simulink model "Ir test"  (R2022a)
settings: Solver=ode3  StartTime=0.0  StopTime=inf  RelTol=1e-3  EnableMultiTasking=on
settings Model: ExtModeTrigDuration=25  Creator=The MathWorks, Inc.  LastModifiedBy=impre
settings SolverCC: AlgebraicLoopSolver=TrustRegion
settings DataIOCC: LimitDataPoints=on  SaveFormat=Array  ReturnWorkspaceOutputs=off
settings OptimizationCC: ExpressionDepthLimit=2147483647  LifeSpan=Inf  MaxStackSize=64
settings DebuggingCC: UnderspecifiedInitializationDetection=Classic  MergeDetectMultiDrivingBlocksExec=none  InheritedTsInSrcMsg=none  FcnCallInpInsideContextMsg=warning  UnconnectedLineMsg=warning  AllowSymbolicDim=off  StateNameClashWarn=warning  SFUnexpectedBacktrackingDiag=warning  SFNoUnconditionalDefaultTransitionDiag=warning  SFExecutionAtInitializationDiag=none  SFMachineParentedDataDiag=warning  ArithmeticOperatorsInVariantConditions=warning
settings HardwareCC: ProdBitPerPointer=32  ProdBitPerSizeT=32  ProdBitPerPtrDiffT=32  ProdLargestAtomicInteger=Long  ProdLargestAtomicFloat=Double  ProdWordSize=32  ProdHWDeviceType=ARM Compatible->ARM Cortex  UseEmbeddedCoderFeatures=off
settings ModelReferenceCC: PropagateSignalLabelsOutOfModel=off
settings SFSimCC: SimUseLocalCustomCode=off  CustomCodeUndefinedFunction=UseInterfaceOnly
settings RTWCC: SystemTargetFile=ert.tlc  HardwareBoard=ARM Cortex-based VEX Microcontroller  TLCOptions=-aInlineSetEventsForThisBaseRateFcn=TLC_FALSE -aSuppressMultiTaskScheduler=TLC_FALSE -aRateBasedStepFcn=0  TemplateMakefile=ert_default_tmf  GenerateReport=on  RTWUseLocalCustomCode=off  Toolchain=GNU Tools for VEX ARM Cortex  LaunchReport=on  DLArmComputeVersion=19.05
settings CodeAppCC: StateflowObjectComments=on
settings ERTTargetCC: CodeReplacementLibrary=GCC ARM Cortex-M3  MultiwordLength=2048  ERTCustomFileBanners=off  SupportContinuousTime=on  SupportNonInlinedSFcns=on  RemoveResetFunc=off  ModelStepFunctionPrototypeControlCompliant=off  ConvertIfToSwitch=off  SuppressUnreachableDefaultCases=off
settings ConfigComp: CovMetricSettings=dw  CovSaveCumulativeToWorkspaceVar=on  CovSaveSingleToWorkspaceVar=on  CovExternalEMLEnable=off  CovSFcnEnable=off

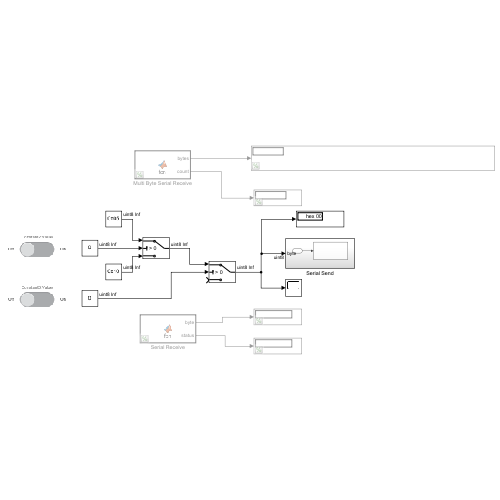
[thumbnail: Simulink's stored preview of the top-level diagram]
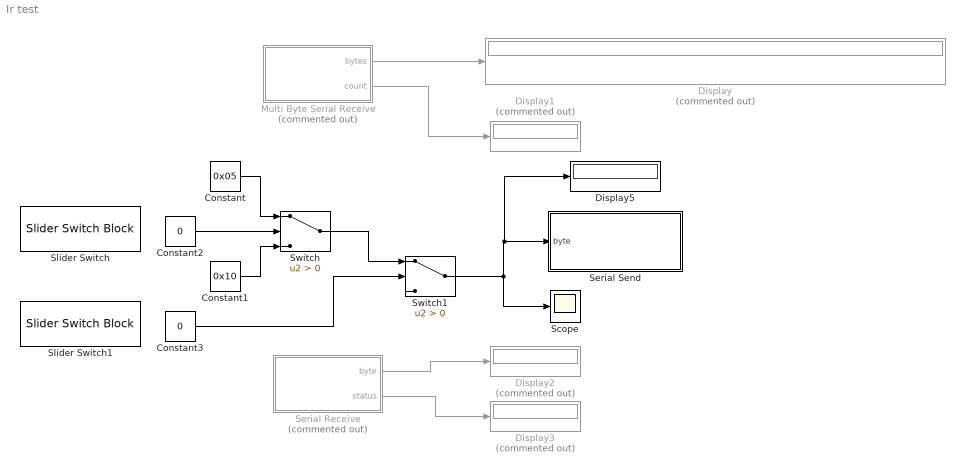
== system Ir test ==
  Constant : Constant  Value=0x05  OutDataTypeStr=uint8
  Constant1 : Constant  Value=0x10  OutDataTypeStr=uint8
  Constant2 : Constant  Value=0  OutDataTypeStr=uint8
  Constant3 : Constant  Value=0  OutDataTypeStr=uint8
  Display{,1..3} (4 alike) : Display  Commented=on
  Display5 : Display
      settings: Format=hex (Stored Integer)
  Multi Byte Serial Receive : MATLAB Function  Commented=on  TreatAsAtomicUnit=on
  Scope : Scope
  Serial Receive : MATLAB Function  Commented=on  TreatAsAtomicUnit=on
  Serial Send : Subsystem
  Slider Switch : SliderSwitchBlock
      settings: Values={{'Off', 'On'}, [0 1]}
  Slider Switch1 : SliderSwitchBlock
      settings: Values={{'Off', 'On'}, [0 1]}
  Switch : Switch  Criteria=u2 > Threshold  SaturateOnIntegerOverflow=off  InputSameDT=off
  Switch1 : Switch  Criteria=u2 > Threshold  SaturateOnIntegerOverflow=off  InputSameDT=off
  wires:
  Multi Byte Serial Receive/1(bytes) -> Display/1
  Multi Byte Serial Receive/2(count) -> Display1/1
  Constant/1 -> Switch/1
  Serial Receive/1(byte) -> Display2/1
  Serial Receive/2(status) -> Display3/1
  Constant1/1 -> Switch/3
  Constant2/1 -> Switch/2
  Switch/1 -> Switch1/1
  Switch1/1 -> Display5/1, Serial Send/1(byte), Scope/1
  Constant3/1 -> Switch1/2

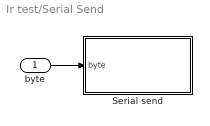
== system Ir test/Serial Send ==
  byte : Inport  OutDataTypeStr=uint8  PortDimensions=[1 1]
  Serial send : MATLAB Function  TreatAsAtomicUnit=on
  wires:
  byte/1 -> Serial send/1(byte)

== matlab function Ir test/Multi Byte Serial Receive ==
  data: bytes output; count output
function [bytes, count] = fcn()
% serial receive
% returns a fixed size array/buffer

%#codegen
persistent isFirstRun
% first "count" bytes correspond to received bytes. rest are kept zero
bufferSize = uint8(50);
count = uint8(0);
bytes = uint8(zeros(1,bufferSize));

if coder.target('Rtw')
    coder.cinclude('API.h');
    coder.cinclude('string.h');
    file = coder.opaque('FILE *', 'uart1','HeaderFile','API.h');

    if isempty(isFirstRun)
        % first time setup
        isFirstRun = false;

        baud = uint32(9600);
        flags = coder.opaque('uint16', 'SERIAL_8N1');
        coder.ceval('usartInit', file, baud, flags);
    end

    coder.ceval('fgets', coder.wref(bytes), bufferSize, file);
    count = coder.ceval('strlen', bytes);
end

end

== matlab function Ir test/Serial Send/Serial send ==
  data: byte input
function fcn(byte)
% Serial send single byte
%#codegen

% Config
port = 'uart1';
baud = uint32(600);

persistent isFirstRun

if coder.target('Rtw')
    coder.cinclude('API.h');
    coder.cinclude('string.h');
    file = coder.opaque('FILE *', port,'HeaderFile','API.h');

    if isempty(isFirstRun)
        % first time setup
        isFirstRun = false;

        flags = coder.opaque('uint16', 'SERIAL_8N1');
        coder.ceval('usartInit', file, baud, flags);
    end

    coder.ceval('fputc', byte, file);

end

end

== matlab function Ir test/Serial Receive ==
  data: byte output; status output
function [byte, status] = fcn()
% serial receive (blocking till a byte is read)
% returns a uint8 byte and status (0 if nothing can be read)

%#codegen

% Config
port = 'uart1';
baud = uint32(600);

persistent isFirstRun
readout = int32(0);
byte = uint8(0);
status = false;

if coder.target('Rtw')
    coder.cinclude('API.h');
    coder.cinclude('string.h');
    file = coder.opaque('FILE *', port,'HeaderFile','API.h');

    if isempty(isFirstRun)
        % first time setup
        isFirstRun = false;

        flags = coder.opaque('uint16', 'SERIAL_8N1');
        coder.ceval('usartInit', file, baud, flags);
    end

    readout = coder.ceval('fgetc', file);
    if readout<0
        byte = uint8(0);
        status = false;
    else
        byte = cast(readout, "uint8");
        status = true;
    end

end

end
